simulink model "lab4model"  (R2021b)
settings: Solver=VariableStepAuto  StartTime=0.0  StopTime=3000  RelTol=1e-6
undefined symbols (not defined in the file): b, C_h, C_w, J, Kt, Kv, L, R, R_ha, R_wh, T_amb, T_nom, T_stall
settings Model: Creator=mluser  LastModifiedBy=mluser

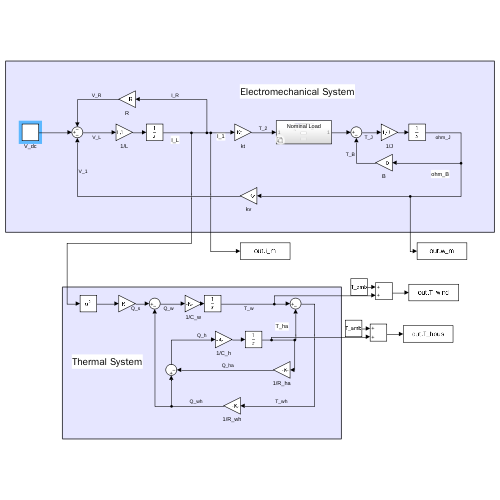
[thumbnail: Simulink's stored preview of the top-level diagram]
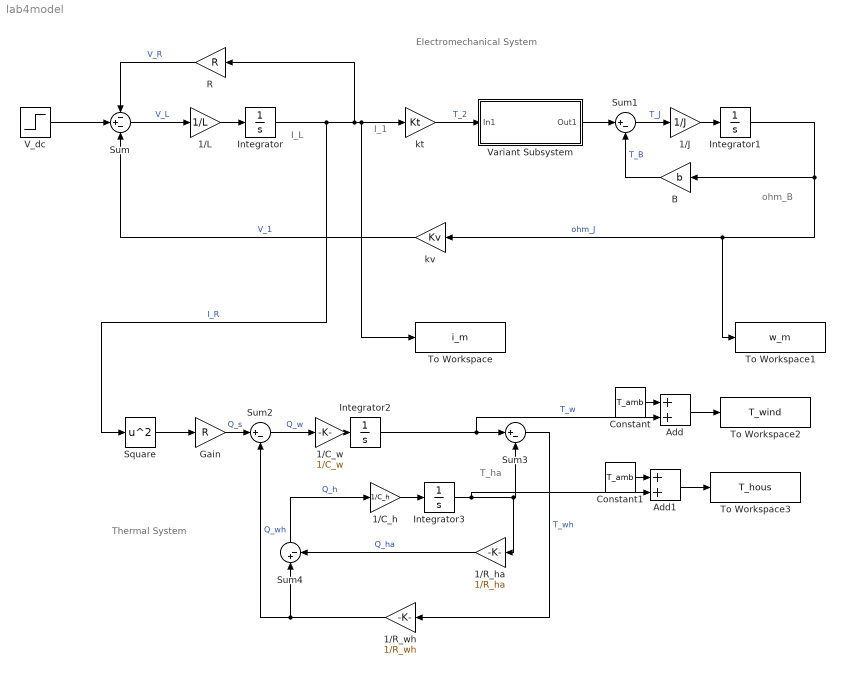
== system lab4model ==
  note: Thermal System
  note: T_ha
  note: Electromechanical System
  note: I_L
  note: ohm_B
  note: I_1
  1/C_h : Gain  Gain=1/C_h
  1/C_w : Gain  Gain=1/C_w
  1/J : Gain  Gain=1/J
  1/L : Gain  Gain=1/L
  1/R_ha : Gain  Gain=1/R_ha
  1/R_wh : Gain  Gain=1/R_wh
  Add : Sum
  Add1 : Sum
  B : Gain  Gain=b
  Constant : Constant  Value=T_amb
  Constant1 : Constant  Value=T_amb
  Gain : Gain  Gain=R
  Integrator{,1..3} (4 alike) : Integrator
  R : Gain  Gain=R
  Square : Math  Operator=square  SaturateOnIntegerOverflow=on
  Sum : Sum  Inputs=-+-
  Sum{1..4} (4 alike) : Sum  Inputs=|+-
  To Workspace : ToWorkspace  VariableName=i_m  SampleTime=-1
  To Workspace1 : ToWorkspace  VariableName=w_m  SampleTime=-1
  To Workspace2 : ToWorkspace  VariableName=T_wind  SampleTime=-1
  To Workspace3 : ToWorkspace  VariableName=T_hous  SampleTime=-1
  V_dc : Step  Time=0  After=18  SampleTime=0
  Variant Subsystem : Subsystem  Variant=on
  kt : Gain  Gain=Kt
  kv : Gain  Gain=Kv
  wires:
  V_dc/1 -> Sum/2
  R/1 -> Sum/1  "V_R"
  kv/1 -> Sum/3  "V_1"
  Sum/1 -> 1/L/1  "V_L"
  1/L/1 -> Integrator/1
  Integrator/1 -> Square/1, R/1, To Workspace/1, kt/1  "I_R"
  kt/1 -> Variant Subsystem/1(In1)  "T_2"
  B/1 -> Sum1/2  "T_B"
  Sum1/1 -> 1/J/1  "T_J"
  1/J/1 -> Integrator1/1
  Integrator1/1 -> B/1, To Workspace1/1, kv/1  "ohm_J"
  Variant Subsystem/1(Out1) -> Sum1/1
  Square/1 -> Gain/1
  Gain/1 -> Sum2/1  "Q_s"
  1/R_wh/1 -> Sum2/2, Sum4/1  "Q_wh"
  Sum3/1 -> 1/R_wh/1  "T_wh"
  1/C_h/1 -> Integrator3/1
  Integrator2/1 -> Add/2, Sum3/1  "T_w"
  Sum2/1 -> 1/C_w/1  "Q_w"
  1/C_w/1 -> Integrator2/1
  Sum4/1 -> 1/C_h/1  "Q_h"
  1/R_ha/1 -> Sum4/2  "Q_ha"
  Constant/1 -> Add/1
  Add/1 -> To Workspace2/1
  Add1/1 -> To Workspace3/1
  Constant1/1 -> Add1/1
  Integrator3/1 -> Add1/2, 1/R_ha/1, Sum3/2

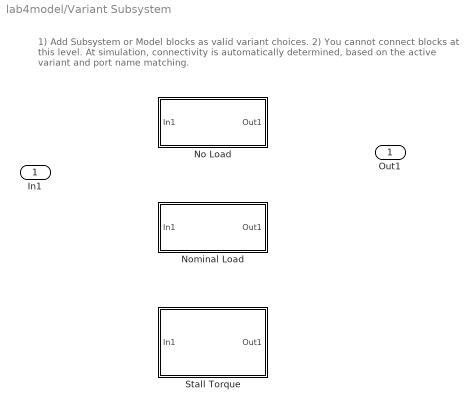
== system lab4model/Variant Subsystem ==
  note: 1) Add Subsystem or Model blocks as valid variant choices.
      | 2) You cannot connect blocks at this level. At simulation, connectivity is automatically
      | determined, based on the active variant and port name matching.
  In1 : Inport
  No Load : Subsystem  VariantControl=T==0
  Nominal Load : Subsystem  VariantControl=T==1
  Stall Torque : Subsystem  VariantControl=T==2
  Out1 : Outport

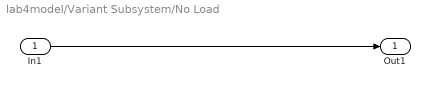
== system lab4model/Variant Subsystem/No Load ==
  In1 : Inport
  Out1 : Outport
  wires:
  In1/1 -> Out1/1

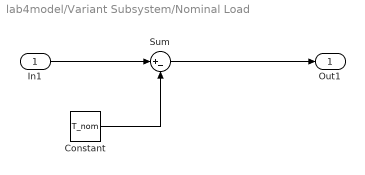
== system lab4model/Variant Subsystem/Nominal Load ==
  In1 : Inport
  Constant : Constant  Value=T_nom
  Sum : Sum  Inputs=|+-
  Out1 : Outport
  wires:
  In1/1 -> Sum/1
  Sum/1 -> Out1/1
  Constant/1 -> Sum/2

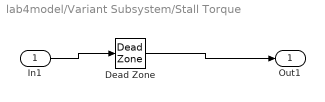
== system lab4model/Variant Subsystem/Stall Torque ==
  In1 : Inport
  Dead Zone : DeadZone  LowerValue=-T_stall  UpperValue=T_stall  SaturateOnIntegerOverflow=on
  Out1 : Outport
  wires:
  In1/1 -> Dead Zone/1
  Dead Zone/1 -> Out1/1
